simulink model "svpwm"  (R2023b)
settings: Solver=FixedStepDiscrete  StartTime=0.0  StopTime=10  FixedStep=Ts  RelTol=1e-3  EnableMultiTasking=on
PreLoadFcn:
  | addpath(pwd);
InitFcn:
  | mc_init;
values from neighbouring files (symbols this model uses):
  Ts = 5e-7    (= 5e-07)    [mc_init.m]
  vd = 0.2 * Udc    (= 19.2)    [mc_init.m]
  vq = 0.2 * Udc    (= 19.2)    [mc_init.m]
settings Model: Creator=kevin  LastModifiedBy=kevin
settings SolverCC: AlgebraicLoopSolver=TrustRegion  AutoInsertRateTranBlk=on
settings DebuggingCC: UnconnectedInputMsg=warning  UnconnectedOutputMsg=warning  UnconnectedLineMsg=warning
settings ModelReferenceCC: EnableRefExpFcnMdlSchedulingChecks=on
settings RTWCC: DLArmComputeVersion=19.05

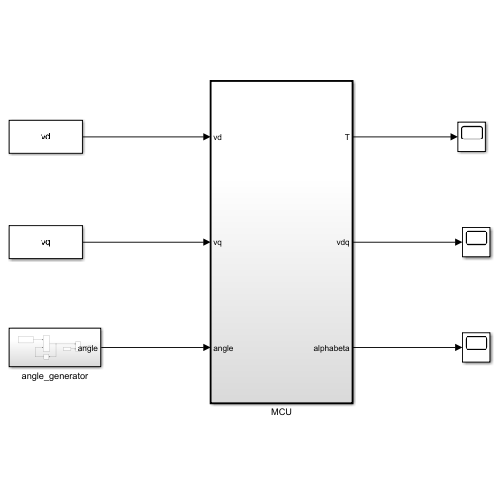
[thumbnail: Simulink's stored preview of the top-level diagram]
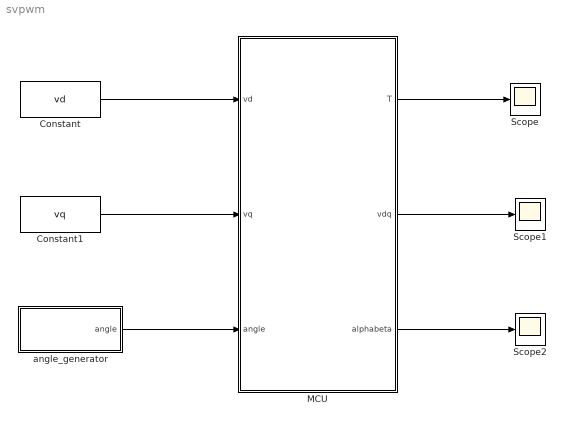
== system svpwm ==
  Constant : Constant  Value=vd
  Constant1 : Constant  Value=vq
  MCU : Subsystem  TreatAsAtomicUnit=on
  Scope : Scope
  Scope1 : Scope
  Scope2 : Scope
  angle_generator : Subsystem
  wires:
  MCU/1(T) -> Scope/1
  Constant/1 -> MCU/1(vd)
  Constant1/1 -> MCU/2(vq)
  angle_generator/1(angle) -> MCU/3(angle)
  MCU/2(vdq) -> Scope1/1
  MCU/3(alphabeta) -> Scope2/1

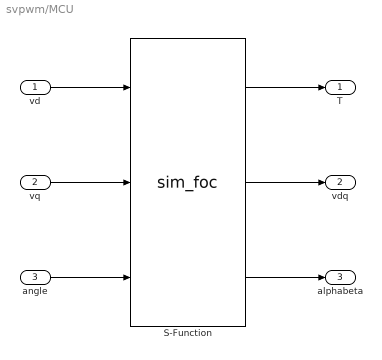
== system svpwm/MCU ==
  vd : Inport
  vq : Inport  Port=2
  angle : Inport  Port=3
  S-Function : S-Function  FunctionName=sim_foc  SFunctionDeploymentMode=off  EnableBusSupport=off
  T : Outport
  vdq : Outport  Port=2
  alphabeta : Outport  Port=3
  wires:
  vd/1 -> S-Function/1
  S-Function/1 -> T/1
  vq/1 -> S-Function/2
  angle/1 -> S-Function/3
  S-Function/2 -> vdq/1
  S-Function/3 -> alphabeta/1

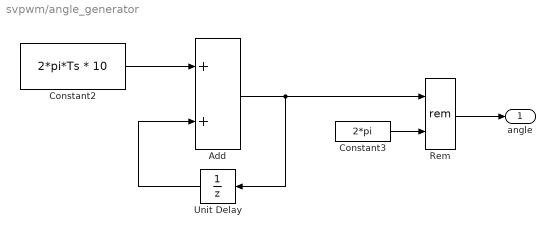
== system svpwm/angle_generator ==
  Add : Sum
  Constant2 : Constant  Value=2*pi*Ts * 10
  Constant3 : Constant  Value=2*pi
  Rem : Math  Operator=rem
  Unit Delay : UnitDelay  SampleTime=-1  HasFrameUpgradeWarning=on
  angle : Outport
  wires:
  Constant2/1 -> Add/1
  Constant3/1 -> Rem/2
  Add/1 -> Unit Delay/1, Rem/1
  Unit Delay/1 -> Add/2
  Rem/1 -> angle/1
